simulink model "RALFCANread"  (R2017b)
settings: Solver=FixedStepAuto  StartTime=0.0  StopTime=inf  FixedStep=0.001  RelTol=1e-3
model workspace (MAT data in the model file):
  SL_ROS_VariableLengthArrays_MaxSizes.CommonInfo.ArrayTruncateAction = 'EmitWarning'
  SL_ROS_VariableLengthArrays_MaxSizes.MsgTypeMap = containers.Map
  SL_ROS_VariableLengthArrays_MaxSizes.MsgTypeMap.serialization.keys = {'std_msgs/Int16MultiArray'}
  SL_ROS_VariableLengthArrays_MaxSizes.MsgTypeMap.serialization.values{1}.PropertyName = 'Data'
  SL_ROS_VariableLengthArrays_MaxSizes.MsgTypeMap.serialization.values{1}.DataType = 'int16'
  SL_ROS_VariableLengthArrays_MaxSizes.MsgTypeMap.serialization.values{1}.MaxLength = 4
  SL_ROS_VariableLengthArrays_MaxSizes.MsgTypeMap.serialization.uniformity = 0
  SL_ROS_VariableLengthArrays_MaxSizes.MsgTypeMap.serialization.keyType = 'char'
  SL_ROS_VariableLengthArrays_MaxSizes.MsgTypeMap.serialization.valueType = 'any'
undefined symbols (not defined in the file): Data, Data_SL_Info
libraries: etargetslib x4, robotlib x2
settings Model: Creator=alf  LastModifiedBy=alf

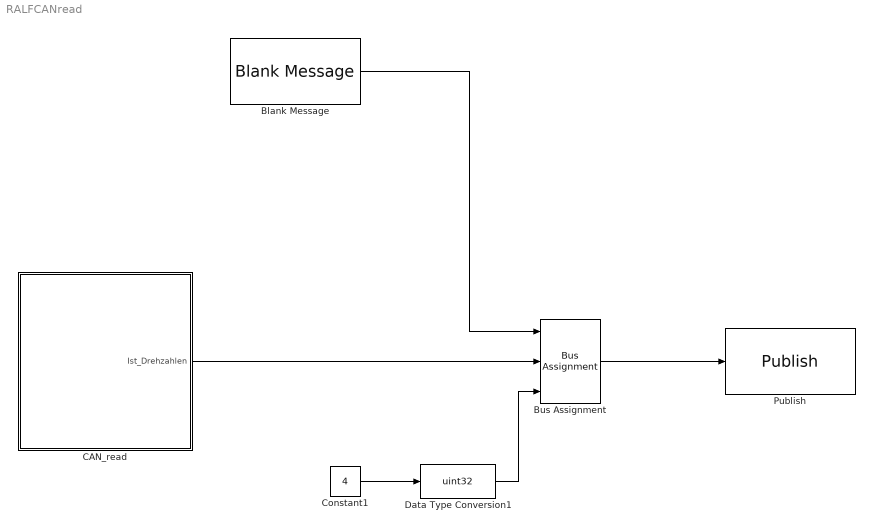
== system RALFCANread ==
  Blank Message : robotlib/Blank Message  SourceLibraryInfo=This block requires Robotics System Toolbox  messageType=std_msgs/Int16MultiArray  SampleTime=inf
      settings: SourceProductBaseCode=RO
  Bus Assignment : BusAssignment  AssignedSignals=Data,Data_SL_Info.CurrentLength
  CAN_read : Subsystem
  Constant1 : Constant  Value=4
  Data Type Conversion1 : DataTypeConversion  OutDataTypeStr=uint32
  Publish : robotlib/Publish  SourceLibraryInfo=This block requires Robotics System Toolbox  topicSource=Specify your own  topic=/CANread  messageType=std_msgs/Int16MultiArray  messageQueueLength=1
      settings: SourceProductBaseCode=RO
  wires:
  Constant1/1 -> Data Type Conversion1/1
  Data Type Conversion1/1 -> Bus Assignment/3
  Blank Message/1 -> Bus Assignment/1
  Bus Assignment/1 -> Publish/1
  CAN_read/1(Ist_Drehzahlen) -> Bus Assignment/2

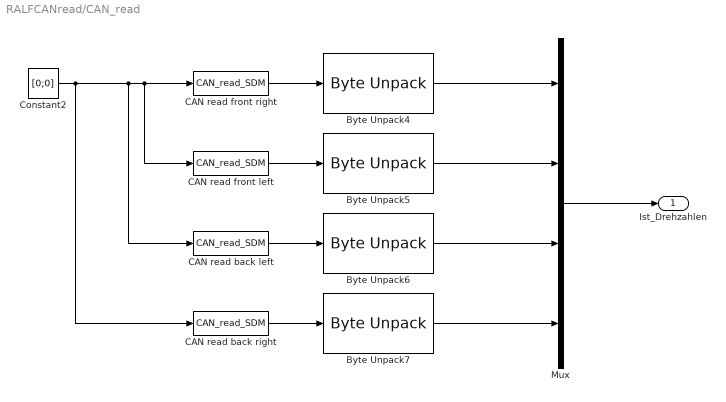
== system RALFCANread/CAN_read ==
  Byte Unpack{4..7} (4 alike) : etargetslib/Byte Unpack  dimensions={[1]}  datatypes={'int16'}  byteAlign=1
  CAN read back left : S-Function  FunctionName=CAN_read_SDM  Parameters=Port,Identifier  SFunctionModules=socketcan  SFunctionDeploymentMode=off  EnableBusSupport=off  mask{Port=can0, Identifier=hex2dec('123')}
      mask prompts: Port "CAN Port"
      mask TypeOptions Port: can0 | can1 | can2
      mask DialogControl DescTextVar Prompt: Dennis Hotze, Dominik Eickmann
  CAN read back right : S-Function  FunctionName=CAN_read_SDM  Parameters=Port,Identifier  SFunctionModules=socketcan  SFunctionDeploymentMode=off  EnableBusSupport=off  mask{Port=can0, Identifier=hex2dec('133')}
      mask prompts: Port "CAN Port"
      mask TypeOptions Port: can0 | can1 | can2
      mask DialogControl DescTextVar Prompt: Dennis Hotze, Dominik Eickmann
  CAN read front left : S-Function  FunctionName=CAN_read_SDM  Parameters=Port,Identifier  SFunctionModules=socketcan  SFunctionDeploymentMode=off  EnableBusSupport=off  mask{Port=can0, Identifier=hex2dec('113')}
      mask prompts: Port "CAN Port"
      mask TypeOptions Port: can0 | can1 | can2
      mask DialogControl DescTextVar Prompt: Dennis Hotze, Dominik Eickmann
  "CAN read front right " : S-Function  FunctionName=CAN_read_SDM  Parameters=Port,Identifier  SFunctionModules=socketcan  SFunctionDeploymentMode=off  EnableBusSupport=off  mask{Port=can0, Identifier=hex2dec('103')}
      mask prompts: Port "CAN Port"
      mask TypeOptions Port: can0 | can1 | can2
      mask DialogControl DescTextVar Prompt: Dennis Hotze, Dominik Eickmann
  Constant2 : Constant  Value=[0;0]
  Mux : Mux
  Ist_Drehzahlen : Outport
  wires:
  "CAN read front right "/1 -> Byte Unpack4/1
  CAN read back left/1 -> Byte Unpack6/1
  CAN read front left/1 -> Byte Unpack5/1
  Constant2/1 -> CAN read back left/1, CAN read front left/1, "CAN read front right "/1, CAN read back right/1
  CAN read back right/1 -> Byte Unpack7/1
  Byte Unpack4/1 -> Mux/1
  Byte Unpack5/1 -> Mux/2
  Byte Unpack6/1 -> Mux/3
  Byte Unpack7/1 -> Mux/4
  Mux/1 -> Ist_Drehzahlen/1
